simulink model "TwoR_Teleoperation_Robust_CAC"  (R2017b)
settings: Solver=ode23s  StartTime=0.0  StopTime=100  MaxStep=0.1  RelTol=1e-7
libraries: simulink x2
settings Model: Creator=ANANDA RANGAN N  LastModifiedBy=ANANDA RANGAN N
settings SolverCC: ZeroCrossAlgorithm=Adaptive  AlgebraicLoopSolver=LineSearch

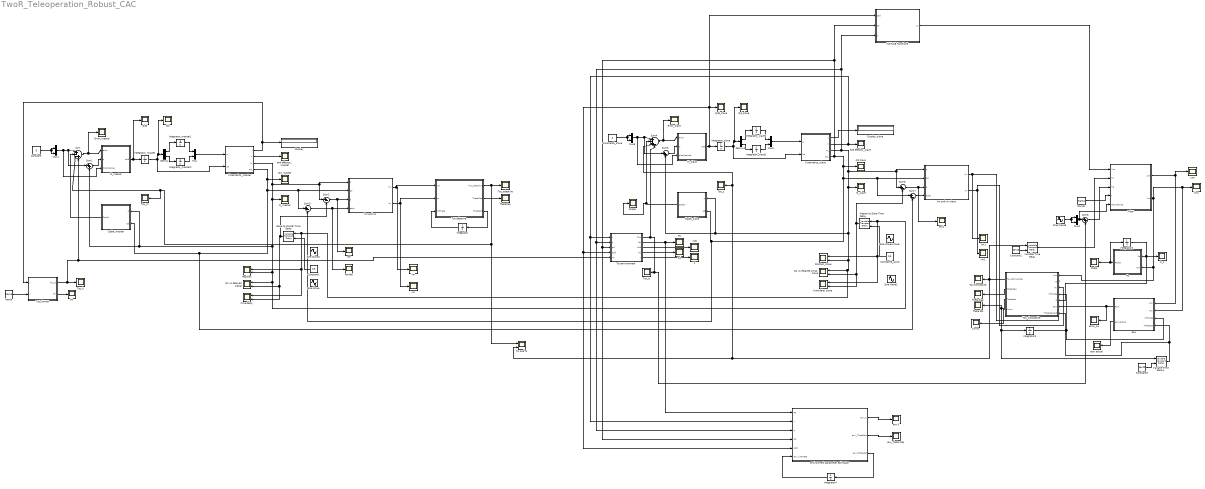
== system TwoR_Teleoperation_Robust_CAC ==
  Constant : Constant  Value=0
  Constant1 : Constant  Value=0.5
  Constant2 : Constant  Value=1e-20
  Constant3 : Constant  Value=1e-20
  Constant5_slave : Constant  Value=0
  Constant6_slave : Constant  Value=0.5
  Cqdot_master : MATLAB Function  TreatAsAtomicUnit=on
  Cqdot_slave : MATLAB Function  TreatAsAtomicUnit=on
  Demux : Demux  Outputs=2
  Demux1 : Demux  Outputs=2
  Display : Display
  Display_slave : Display
  Error_master : Scope
  Fe : Scope
  Fh : Scope
  Filter : MATLAB Function  TreatAsAtomicUnit=on
  Integrator : Integrator
  Integrator2 : Integrator  InitialCondition=[1 0 0; 0 1 0; 0 0 1]
  Integrator3 : Integrator
  Integrator4 : Integrator
  Integrator_master : Integrator
  Integrator_master1 : Integrator  InitialCondition=pi/2
  Integrator_master2 : Integrator
  Integrator_slave : Integrator
  Integrator_slave1 : Integrator  InitialCondition=pi/2
  Integrator_slave2 : Integrator
  Kinematics_master : MATLAB Function  TreatAsAtomicUnit=on
  Kinematics_slave : MATLAB Function  TreatAsAtomicUnit=on
  Kmrm : Scope
  MATLAB Function3 : MATLAB Function  TreatAsAtomicUnit=on
  M_master : MATLAB Function  TreatAsAtomicUnit=on
  M_slave : MATLAB Function  TreatAsAtomicUnit=on
  Master to Slave Time Delay : VariableTransportDelay  MaximumDelay=10
  Mux{,1..2,5..6} (5 alike) : Mux  Inputs=2
  P_s : Scope
  Position : Scope  NumInputPorts=2
  Position_slave : Scope  NumInputPorts=2
  Ps : MATLAB Function  TreatAsAtomicUnit=on
  Psdot : Scope
  Q_master : Scope
  Q_slave : Scope
  Qd : Scope
  Qd slave : Scope
  Qd_master : Scope
  Qd_slave : Scope
  Qdd : Scope
  Qdd_slave : Scope
  Qs vs delayed signal : Scope  NumInputPorts=2
  Qs vs delayed signal slave : Scope  NumInputPorts=2
  Ramp : simulink/Sources/Ramp  slope=1  start=0  X0=0
  Ramp1 : simulink/Sources/Ramp  slope=1  start=0  X0=0
  Scope : Scope
  Sine Wave : Sin  Amplitude=0.5  Bias=0.5  Phase=3*pi/2  SampleTime=0
  Sine Wave1 : Sin  Amplitude=0.5  Bias=1  SampleTime=0
  Sine Wave1 slave : Sin  Amplitude=0.5  Bias=1  SampleTime=0
  Sine Wave2 : Sin  Amplitude=0.5  Bias=0.5  Phase=3*pi/2  SampleTime=0
  Sine Wave3 : Sin  Amplitude=2  Frequency=100  SampleTime=0
  Slave to Master Time Delay : VariableTransportDelay  MaximumDelay=10
  Sum : Sum  Inputs=|+--+
  Sum1 : Sum  Inputs=|++
  Sum{2..3,6..7} (4 alike) : Sum  Inputs=|+-
  Sum4 : Sum  Inputs=|+-+-
  Sum5 : Sum  Inputs=|++
  Sum8 : Sum  Inputs=|++
  Theta Cap : Scope
  Theta dot : Scope
  ThetaCap : Scope
  Tm and Ts : Scope  NumInputPorts=2
  Tou Composite : Scope
  Tou adaptive : MATLAB Function  TreatAsAtomicUnit=on
  Tou environment : MATLAB Function  TreatAsAtomicUnit=on
  Tou_Composite : MATLAB Function  TreatAsAtomicUnit=on
  Tou_adaptive : Scope
  Tou_e : Scope
  Tou_h : Scope
  Tou_human : MATLAB Function  TreatAsAtomicUnit=on
  Tou_m : Scope
  Tou_s : Scope
  Variable Time Delay : VariableTransportDelay  MaximumDelay=10
  Variable Time Delay1 : VariableTransportDelay  MaximumDelay=10
  X : Scope
  Xd : Scope
  Xdd : Scope
  Ym : Scope
  Ym and rm : MATLAB Function  TreatAsAtomicUnit=on
  Ym and rm slave : MATLAB Function  TreatAsAtomicUnit=on
  Ym1 : Scope
  Ysw : Scope
  em : Scope
  em1 : Scope
  emdot : Scope
  end effector_master : Scope
  end effector_slave : Scope
  env K : Scope
  env_Theta Cap : Scope
  environment parameter estimator : MATLAB Function  TreatAsAtomicUnit=on
  error_slave : Scope
  error_sw : Scope
  esw : MATLAB Function  TreatAsAtomicUnit=on
  esw actual : Scope
  rm : Scope
  rm1 : Scope
  time delay : Scope  NumInputPorts=2
  time delay slave : Scope  NumInputPorts=2
  ysw : Scope
  wires:
  M_master/1(qdd) -> Qdd/1, Integrator_master/1
  Integrator_master/1 -> Qd/1, Demux/1, Kinematics_master/2(qd)
  Demux/1 -> Integrator_master1/1
  Demux/2 -> Integrator_master2/1
  Integrator_master1/1 -> Mux/1
  Integrator_master2/1 -> Mux/2
  Mux/1 -> Kinematics_master/1(q)
  Constant/1 -> Mux1/1, Mux1/2
  Mux1/1 -> M_master/3(disturbance), Sum/1, Sum1/1
  Cqdot_master/1(Cqdot) -> Sum/2
  Tou adaptive/1(Tou_adaptive) -> Tm and Ts/1, Tou_m/1, Sum/3, Tou_adaptive/1
  Sum1/1 -> M_master/2(q)
  Sum/1 -> Error_master/1, M_master/1(error)
  Kinematics_master/1(J) -> Display/1, Tou_human/1(J)
  Slave to Master Time Delay/1 -> Qs vs delayed signal/2, time delay/2, Sum2/2
  Constant1/1 -> Slave to Master Time Delay/2
  Sum2/1 -> em/1, Ym and rm/3(e)
  Ym and rm/1(Ym) -> Tou adaptive/1(Ym), Ym/1
  Ym and rm/2(rm) -> Tou adaptive/2(rm), rm/1
  Tou adaptive/3(Thetadot) -> Integrator/1
  Integrator/1 -> Tou adaptive/3(intTheta)
  Tou adaptive/2(ThetaCap) -> ThetaCap/1
  Sum3/1 -> emdot/1, Ym and rm/4(edot)
  Integrator_slave1/1 -> Mux5/1
  Kinematics_master/3(q_) -> Sum2/1, Ym and rm/1(q), Q_master/1, Position/2, Master to Slave Time Delay/1, Position_slave/1, time delay slave/1, Qs vs delayed signal/1, Sum1/2, Cqdot_master/1(q)
  Kinematics_master/4(qd_) -> Ym and rm/2(qd), Sum3/1, Sum7/2, Cqdot_master/2(qd), Qd_master/1
  Constant6_slave/1 -> Master to Slave Time Delay/2
  Ym and rm slave/1(Ym) -> Tou_Composite/2(Ys), Ym1/1
  Mux5/1 -> Kinematics_slave/1(q)
  Sum6/1 -> em1/1, Ym and rm slave/3(e)
  Master to Slave Time Delay/1 -> Qs vs delayed signal slave/2, time delay slave/2, Sum6/2
  Kinematics_slave/1(J) -> Display_slave/1
  Cqdot_slave/1(Cqdot) -> Scope/1, Sum4/2
  Constant5_slave/1 -> Mux6/1, Mux6/2
  Demux1/1 -> Integrator_slave1/1
  Kinematics_slave/4(qd_) -> Ym and rm slave/2(qd), Sum7/1, Sum3/2, Cqdot_slave/2(qd), Qd slave/1, environment parameter estimator/4(qd), Tou environment/3(qd), MATLAB Function3/2(qd)
  Sum5/1 -> M_slave/2(q)
  Demux1/2 -> Integrator_slave2/1
  Integrator_slave2/1 -> Mux5/2
  Sum4/1 -> error_slave/1, M_slave/1(error)
  Integrator_slave/1 -> Qd_slave/1, Demux1/1, Kinematics_slave/2(qd)
  Sum7/1 -> Ym and rm slave/4(edot)
  Ym and rm slave/2(rm) -> Tou_Composite/3(rm), rm1/1
  Tou environment/3(Xdd) -> Xdd/1
  Tou environment/4(Xd) -> Xd/1
  Tou environment/5(x) -> X/1
  Ramp/1 -> Tou_human/2(t)
  Kinematics_master/2(X) -> end effector_master/1
  Tou_human/2(Fh) -> Fh/1
  Ramp1/1 -> Filter/4(t)
  Filter/1(ysw) -> ysw/1, esw/1(ysw)
  Filter/2(Ysw) -> esw/2(Ysw), Ysw/1, Tou_Composite/1(Ysw), Ps/2(Ysw)
  Ps/1(Psdot) -> Psdot/1, Integrator2/1
  Integrator2/1 -> Tou_Composite/5(P), P_s/1, Ps/1(Ps)
  esw/1(esw) -> error_sw/1, Tou_Composite/6(esw)
  Integrator3/1 -> esw/3(intTheta), Tou_Composite/4(intTheta)
  Tou_Composite/2(ThetaCap) -> Theta Cap/1
  Tou_Composite/1(Tou_Composite) -> Variable Time Delay/1, Tou Composite/1, Tou_s/1, Sum4/3, Tm and Ts/2
  Variable Time Delay/1 -> Filter/2(Ts)
  Constant2/1 -> Variable Time Delay/2
  Tou_human/1(Tou_h) -> Tou environment/5(Th), Sum/4, Tou_h/1
  Tou_Composite/4(Kmrm) -> Kmrm/1
  MATLAB Function3/1(Ys) -> Filter/1(Yso)
  esw/2(esw_actual) -> esw actual/1
  Tou environment/1(Tou) -> Sum8/2, Tou_e/1, Sum4/4
  Tou_Composite/3(Thetadot) -> Theta dot/1, Variable Time Delay1/1, Integrator3/1
  Constant3/1 -> Variable Time Delay1/2
  Variable Time Delay1/1 -> Tou_Composite/7(Thetadot_old), esw/4(Thetadot)
  Sum8/1 -> Filter/3(Te)
  Sine Wave3/1 -> Mux2/2, Mux2/1
  Mux2/1 -> Filter/5(disturbance), Sum8/1
  Tou environment/2(Fe) -> environment parameter estimator/1(Fe), Fe/1
  Kinematics_slave/3(q_) -> Sum6/1, Ym and rm slave/1(q), Q_slave/1, Position_slave/2, Position/1, time delay/1, Slave to Master Time Delay/1, Qs vs delayed signal slave/1, Sum5/2, Cqdot_slave/1(q), Tou environment/2(q), environment parameter estimator/3(q), MATLAB Function3/3(q)
  Kinematics_slave/2(X) -> environment parameter estimator/2(x), Tou environment/1("x "), end effector_slave/1
  M_slave/1(qdd) -> MATLAB Function3/1(qdd), Qdd_slave/1, Tou environment/4(qdd), environment parameter estimator/5(qdd), Integrator_slave/1
  environment parameter estimator/3(env_Thetadot) -> Integrator4/1
  Integrator4/1 -> environment parameter estimator/6(env_intTheta)
  environment parameter estimator/2(env_ThetaCap) -> env_Theta Cap/1
  environment parameter estimator/1(env_K) -> env K/1
  Mux6/1 -> M_slave/3(disturbance), Sum4/1, Sum5/1

== matlab function TwoR_Teleoperation_Robust_CAC/M_master ==
  data: error input; qdd output; q input; disturbance input
function qdd = fcn(error, q, disturbance)

q1 = q(1);
q2 = q(2);

m1 = 0.5;
m2 = 0.5;

l = 0.3;

M = [(m1+m2)*l*l + m2*l*l + 2*m2*l*l*cos(q2), m2*l*l + m2*l*l*cos(q2);
      m2*l*l + m2*l*l*cos(q2), m2*l*l];
  
Minv = inv(M);

qdd = Minv*(error-disturbance);

== matlab function TwoR_Teleoperation_Robust_CAC/Cqdot_master ==
  data: q input; Cqdot output; qd input
function Cqdot = fcn(q, qd)

q1 = q(1);
q2 = q(2);

qd1 = qd(1);
qd2 = qd(2);

l =0.5;
m1 = 0.5;
m2 = 0.5;

C11 = -2*l*l*m2*sin(q2)*qd2;
C12 = -l*l*m2*sin(q2)*qd2;
C21 = m2*l*l*sin(q2)*qd1;
C22 = 0;

C = [C11, C12;
     C21, C22];
 
Cqdot = C*qd;
Cqdot = [0;0];

== matlab function TwoR_Teleoperation_Robust_CAC/Kinematics_master ==
  data: q input; J output; qd input; X output; q_ output; qd_ output
function [J, X, q_, qd_] = fcn(q, qd)

q1 = q(1);
q2 = q(2);

qd1 = qd(1);
qd2 = qd(2);

dt = 1e-9;

l = 0.3;
%
if q1<0.05
    q1 = 0.05;
    qd1 = 0;
else if q1>(pi-0.05)
        q1 = (pi-0.05);
        qd1 = 0;
    end
end
if q2<0.01
    q2 = 0.01;
    qd2 = 0;
else if q2>(pi-0.01)
        q2 = (pi-0.01);
        qd2 = 0;
    end
end
%

X = [0;0];

x = l*(cos(q1) + cos(q1+q2));
y = l*(sin(q1) + sin(q1+q2));

X = [x; y];

dx1 = -l*(sin(q1) + sin(q1+q2));
dy1 = l*(cos(q1) + cos(q1+q2));
dx2 = -l*cos(q1+q2);
dy2 = l*sin(q1+q2);

J = [dx1 dx2;
     dy1 dy2];
 
q_ = [q1; q2];
qd_ = [qd1; qd2];

== matlab function TwoR_Teleoperation_Robust_CAC/Ym and rm ==
  data: q input; Ym output; qd input; e input; edot input; rm output
function [Ym, rm] = fcn(q, qd, e, edot)

q1 = q(1);
q2 = q(2);

qd1 = qd(1);
qd2 = qd(2);

lambda = 5;

Ym = [(lambda*edot(1)), lambda*((2*edot(1)*cos(q2))+(edot(2)*cos(q2))-(sin(q2)*qd2*e(1))-(sin(q2)*(qd1+qd2)*e(2))), lambda*edot(2);
      0 lambda*((cos(q2)*edot(1))+(sin(q2)*qd1*e(1))) lambda*(edot(1)+edot(2))];
 
rm = 2.5*qd + (lambda*e);

== matlab function TwoR_Teleoperation_Robust_CAC/Tou adaptive ==
  data: Ym input; Tou_adaptive output; rm input; intTheta input; ThetaCap output; Thetadot output
function [Tou_adaptive, ThetaCap, Thetadot] = fcn(Ym, rm, intTheta)

Km = 5*[1 0 ; 0 1];   
T = 0.05*[1 0 0; 0 1 0 ; 0 0 1]; 

m1 = 1.5;
m2 = 0.75;

l = 0.4 ;

alpha = m2*l*l + (m1+m2)*l*l;
beta = m2*l*l;
delta = m2*l*l;

Theta_initial = [alpha; beta; delta];
ThetaCap = Theta_initial + intTheta;

Tou_adaptive = 0.01*Ym*ThetaCap + Km*rm;
Thetadot = T*(Ym')*rm;

== matlab function TwoR_Teleoperation_Robust_CAC/Cqdot_slave ==
  data: q input; Cqdot output; qd input
function Cqdot = fcn(q, qd)

q1 = q(1);
q2 = q(2);

qd1 = qd(1);
qd2 = qd(2);

m1 = 1.5;
m2 = 0.75;

l = 0.4 ;

C11 = -2*l*l*m2*sin(q2)*qd2;
C12 = -l*l*m2*sin(q2)*qd2;
C21 = m2*l*l*sin(q2)*qd1;
C22 = 0;

C = [C11, C12;
     C21, C22];
 
Cqdot = C*qd;

== matlab function TwoR_Teleoperation_Robust_CAC/Kinematics_slave ==
  data: q input; J output; qd input; X output; q_ output; qd_ output
function [J, X, q_, qd_] = fcn(q, qd)

q1 = q(1);
q2 = q(2);

qd1 = qd(1);
qd2 = qd(2);


l = 0.3;
%
if q1<0.01
    q1 = 0.01;
else if q1>(pi-0.01)
        q1 = (pi-0.01);
    end
end
if q2<0.01
    q2 = 0.01;
else if q2>(pi-0.01)
        q2 = (pi-0.01);
    end
end
%
X = [0;0];

x = l*(cos(q1) + cos(q1+q2));
y = l*(sin(q1) + sin(q1+q2));

X = [x; y];

dx1 = -l*(sin(q1) + sin(q1+q2));
dy1 = l*(cos(q1) + cos(q1+q2));
dx2 = -l*sin(q1+q2);
dy2 = l*cos(q1+q2);

J = [dx1 dx2;
     dy1 dy2];

q_ = [q1; q2];
qd_ = [qd1; qd2];

== matlab function TwoR_Teleoperation_Robust_CAC/M_slave ==
  data: error input; qdd output; q input; disturbance input
function qdd = fcn(error, q, disturbance)

q1 = q(1);
q2 = q(2);

m1 = 1.5;
m2 = 0.75;

l = 0.4 ;

M = [(m1+m2)*l*l + m2*l*l + 2*m2*l*l*cos(q2), m2*l*l + m2*l*l*cos(q2);
      m2*l*l + m2*l*l*cos(q2), m2*l*l];
  
Minv = inv(M);

qdd = Minv*(error-disturbance);

== matlab function TwoR_Teleoperation_Robust_CAC/Ym and rm slave ==
  data: q input; Ym output; qd input; e input; edot input; rm output
function [Ym, rm] = fcn(q, qd, e, edot)

q1 = q(1);
q2 = q(2);

qd1 = qd(1);
qd2 = qd(2);

lambda = 5;

Ym = [(lambda*edot(1)), lambda*((2*edot(1)*cos(q2))+(edot(2)*cos(q2))-(sin(q2)*qd2*e(1))-(sin(q2)*(qd1+qd2)*e(2))), lambda*edot(2);
      0 lambda*((cos(q2)*edot(1))+(sin(q2)*qd1*e(1))) lambda*(edot(1)+edot(2))];
 
rm = 5*qd + (lambda*e);

== matlab function TwoR_Teleoperation_Robust_CAC/Tou environment ==
  data: x input; Tou output; q input; qd input; qdd input; Fe output; Xdd output; Xd output; x output; Th input
function [Tou, Fe, Xdd, Xd, x]  = fcn(x, q, qd, qdd, Th)

q1 = q(1);
q2 = q(2);

l = 0.3;

dx1 = -l*(sin(q1) + sin(q1+q2));
dy1 = l*(cos(q1) + cos(q1+q2));
dx2 = -l*sin(q1+q2);
dy2 = l*cos(q1+q2);

J = [dx1 dx2;
     dy1 dy2];
 
Xd = J*qd;

ddx1 = -l*(cos(q1) + cos(q1+q2));
ddy1 = -l*(sin(q1) + sin(q1+q2));
ddx2 = -l*cos(q1+q2);
ddy2 = -l*sin(q1+q2);

Jdot = [ddx1 ddx2;
        ddy1 ddy2];

Xdd = (J*qdd) + (Jdot*qd);

Fh = inv(J')*Th;

Fe = [0;0];
%
if x(1) >= 0
    Fe(1) = 20000*(x(1)) + 200*Xd(1);% + 50*Xdd(1);
else if x(1) == 0.4
       Fe = Fh;
    else
        Fe(1) = 0;
    end
end
%
Tou = (J')*Fe;

== matlab function TwoR_Teleoperation_Robust_CAC/Tou_human ==
  data: J input; t input; Tou_h output; Fh output
function [Tou_h, Fh] = fcn(J, t)
Tou_h = [0;0];
Fh = [0;0];
%{
if t < 15
    Tou_h(1) = -1;
else if t < 39
        Tou_h(1) = -(t/3);
    else
        Tou_h(1) = -15;
    end
end
%}
%{
if t>5 && t<10
    Fh(1) = 2;
else if t>10 && t<15
        Fh(1) = (-0.4*t) + 6;
    else if t>20 && t<25
         Fh(1) = 5;
        else if t>25 && t<30
                Fh(1) = -t + 30;
            else
                Fh(1) = 0;
            end
        end
    end
end
%}
%
if t>5
    Fh(1) = 5;
end
%
%{
if t>5 && t<10
    Fh(1) = 20;
else Fh(1) = 0;
%else if t>10 && t<15
%        Fh(1) = -(2*t) + 30; 
%    end
end
%}
Tou_h = (J')*Fh;

== matlab function TwoR_Teleoperation_Robust_CAC/Filter ==
  data: Yso input; Ts input; Te input; ysw output size=[2]; t input; Ysw output size=[2 3]; disturbance input
function [ysw, Ysw] = fcn(Yso, Ts, Te, t, disturbance)
%{
w = 5.5*exp(-5.5*t);

ysw = conv(w,Tf);

Y1 = [0,0,0];
Y1(1) = Yso(1);
Y1(2) = Yso(2);
Y1(3) = Yso(3);

Y1 = conv(w, Y1);

Y1(1) = Yso(4);
Y1(2) = Yso(5);
Y1(3) = Yso(6);

Y2 = conv(w,Y1);

Ysw = [Y1; Y2];
%}

ysw = Ts - (Te - disturbance);
Ysw = Yso;

== matlab function TwoR_Teleoperation_Robust_CAC/Ps ==
  data: Ps input; Psdot output; Ysw input
function Psdot = fcn(Ps, Ysw)

Psdot = -10*Ps*(Ysw')*Ysw*Ps;

== matlab function TwoR_Teleoperation_Robust_CAC/esw ==
  data: ysw input; esw output; Ysw input; intTheta input; esw_actual output; Thetadot input
function [esw, esw_actual] = fcn(ysw, Ysw, intTheta, Thetadot)

m1 = 1.5;
m2 = 0.75;

l = 0.4 ;

alpha = m2*l*l + (m1+m2)*l*l;
beta = m2*l*l;
delta = m2*l*l;

Theta_initial = [0;0;0];
Theta_correct = [alpha; beta; delta];
ThetaCap = Theta_initial + intTheta;

esw = [0;0];
%esw = (Ysw*((10^5)*(Theta_correct - ThetaCap) + 0.005*Thetadot));
esw = (10^5)*(ysw - Ysw*ThetaCap);

esw_actual = ysw - Ysw*Theta_correct ;

== matlab function TwoR_Teleoperation_Robust_CAC/Tou_Composite ==
  data: Ysw input; Tou_Composite output; Ys input; rm input; intTheta input; ThetaCap output; Thetadot output; P input; esw input; Kmrm output; Thetadot_old input
function [Tou_Composite, ThetaCap, Thetadot, Kmrm] = fcn(Ysw, Ys, rm, intTheta, P, esw, Thetadot_old)
Km = 5*[1 0 ; 0 1];   
KdeltaM = 0.5*[1 0;0 1];

m1 = 1.5;
m2 = 0.75;

l = 0.4 ;

alpha = m2*l*l + (m1+m2)*l*l;
beta = m2*l*l;
delta = m2*l*l;

Theta_initial = [0;0;0];
ThetaCap = Theta_initial + intTheta;

sig = sign(rm);

if abs(rm(1)) < 1
    sig(1) = (rm(1));
end

if abs(rm(2)) < 1
    sig(2) = (rm(2));
end

Tou_Composite = -Ys*ThetaCap - Km*rm - KdeltaM*(sig);
Kmrm = Km*rm;
Thetadot = [0;0;0];
%Thetadot = P*((Ysw')*esw +(Ys')*rm);

T = [100 0 0; 0 100 0; 0 0 100];
Thetadot = ((Ysw')*esw +(Ys')*rm);

== matlab function TwoR_Teleoperation_Robust_CAC/MATLAB Function3 ==
  data: qdd input; qd input; q input; Ys output
function Ys = fcn(qdd, qd, q)

q1 = q(1); q2 = q(2);
qd1 = qd(1); qd2 = qd(2);
qdd1 = qdd(1); qdd2 = qdd(2);


Y12 = (2*cos(q2)*qdd1) + (cos(q2)*qdd2) - (2*sin(q2)*qd1*qd2) - (sin(q2)*qd2*qd2);
Y22 = (cos(q2)*qdd1) + sin(q2)*qd1*qd1;

Ys = [qdd(1), Y12, qdd(2);
      0, Y22, qdd(1)+qdd(2)];

== matlab function TwoR_Teleoperation_Robust_CAC/environment parameter estimator ==
  data: Fe input; x input; q input; qd input; env_K output; env_ThetaCap output; qdd input; env_intTheta input; env_Thetadot output
function [env_K, env_ThetaCap, env_Thetadot] = fcn(Fe, x, q, qd, qdd, env_intTheta)

l = 0.3;
q1 = q(1);
q2 = q(2);

T = 500*[1 0 0; 0 1 0; 0 0 1];
T2 = [1e6 0; 0 1e4];
T8 = 500;

dx1 = -l*(sin(q1) + sin(q1+q2));
dy1 = l*(cos(q1) + cos(q1+q2));
dx2 = -l*sin(q1+q2);
dy2 = l*cos(q1+q2);

J = [dx1 dx2;
     dy1 dy2];

xd = J*qd;

ddx1 = -l*(cos(q1) + cos(q1+q2));
ddy1 = -l*(sin(q1) + sin(q1+q2));
ddx2 = -l*cos(q1+q2);
ddy2 = -l*sin(q1+q2);

Jdot = [ddx1 ddx2;
        ddy1 ddy2];

xdd = (Jdot*qd) + (J*qdd);

%{
env_Y = [ xd(1) x(1);
          xd(2) x(2)];
     
env_Theta_initial = [0;0];

env_ThetaCap = env_Theta_initial + env_intTheta;

Fe_Cap = env_Y*env_ThetaCap;

env_Thetadot = -T2*(env_Y')*(Fe_Cap-Fe);
%}
env_K = [Fe(1)/x(1);Fe(2)/x(2)];


env_Y = [x(1) xd(1)];

env_Theta_initial = [0;0];

env_ThetaCap = env_Theta_initial + env_intTheta;

Fe_Cap = (env_Y)*(env_ThetaCap);

env_Thetadot = -(T2)*(env_Y')*(Fe_Cap-Fe(1));
